simulink model "TENNIS_Ball"  (R2017a)
settings: Solver=ode4  StartTime=0.0  StopTime=1.5  FixedStep=.01  RelTol=1e-7  EnableMultiTasking=on
InitFcn:
  | h =1;        % [m];
  | v0=25;      % [m*s^-1];
  | theta=15;  % [deg];
  | ro=1.29;    % [kg*m^-3];
  | g=9.81;     % [m/s^2]
  | d=.063;     % [m];
  | m=.05;      % [kg];
  | w=20;        % [m*s^-1]; angular velocity of a spinning ball
  | eta=1;        % describes direction(+-) and presence of rotation;
settings Model: Creator=SLE  LastModifiedBy=sulaymon.eshkabilov
settings DataIOCC: Decimation=4  SignalLoggingSaveFormat=ModelDataLogs  SignalLogging=off  SaveTime=off  ReturnWorkspaceOutputs=on
settings OptimizationCC: ExpressionDepthLimit=2147483647  LifeSpan=inf
settings DebuggingCC: UnderspecifiedInitializationDetection=Classic  MergeDetectMultiDrivingBlocksExec=none  SolverPrmCheckMsg=warning  FcnCallInpInsideContextMsg=warning  StateNameClashWarn=warning  SFUnexpectedBacktrackingDiag=warning  SFNoUnconditionalDefaultTransitionDiag=warning  SFExecutionAtInitializationDiag=none
settings HardwareCC: ProdBitPerPointer=32  ProdBitPerSizeT=32  ProdBitPerPtrDiffT=32  ProdLargestAtomicFloat=None  ProdIntDivRoundTo=Undefined  ProdEndianess=Unspecified  ProdWordSize=32  ProdHWDeviceType=32-bit Generic
settings ModelReferenceCC: PropagateSignalLabelsOutOfModel=off
settings RTWCC: GenCodeOnly=on  GenerateReport=on  TLCDebug=on  TLCAssert=on  RTWUseSimCustomCode=on  LaunchReport=on  TargetLang=C++
settings CodeAppCC: ForceParamTrailComments=on  UseSimReservedNames=on
settings GRTTargetCC: TargetLangStandard=C89/C90 (ANSI)  GeneratePreprocessorConditionals=Disable all  CombineOutputUpdateFcns=off  GRTInterface=on
settings ConfigComp: CovMetricSettings=dw  CovHtmlReporting=on  CovSaveCumulativeToWorkspaceVar=on  CovSaveSingleToWorkspaceVar=on  CovExternalEMLEnable=off

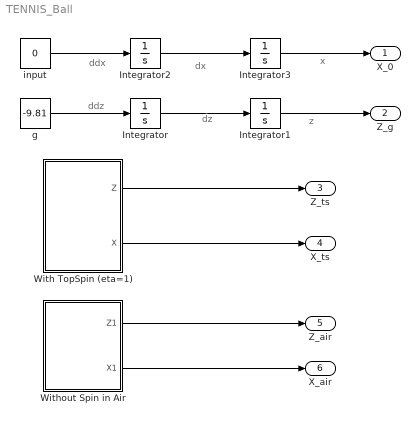
== system TENNIS_Ball ==
  note: dx
  note: x
  note: dz
  note: ddz
  note: z
  note: ddx
  Integrator : Integrator  InitialCondition=25*sin(15*pi/180)
  Integrator1 : Integrator  InitialCondition=1
  Integrator2 : Integrator  InitialCondition=25*cos(15*pi/180)
  Integrator3 : Integrator
  With TopSpin (eta=1) : Subsystem
  Without Spin in Air : Subsystem
  g : Constant  Value=-9.81
  input : Constant  Value=0
  X_0 : Outport
  Z_g : Outport  Port=2
  Z_ts : Outport  Port=3
  X_ts : Outport  Port=4
  Z_air : Outport  Port=5
  X_air : Outport  Port=6
  wires:
  Integrator/1 -> Integrator1/1
  Integrator1/1 -> Z_g/1
  Integrator2/1 -> Integrator3/1
  Integrator3/1 -> X_0/1
  g/1 -> Integrator/1
  input/1 -> Integrator2/1
  With TopSpin (eta=1)/1(Z) -> Z_ts/1
  With TopSpin (eta=1)/2(X) -> X_ts/1
  Without Spin in Air/1(Z1) -> Z_air/1
  Without Spin in Air/2(X1) -> X_air/1

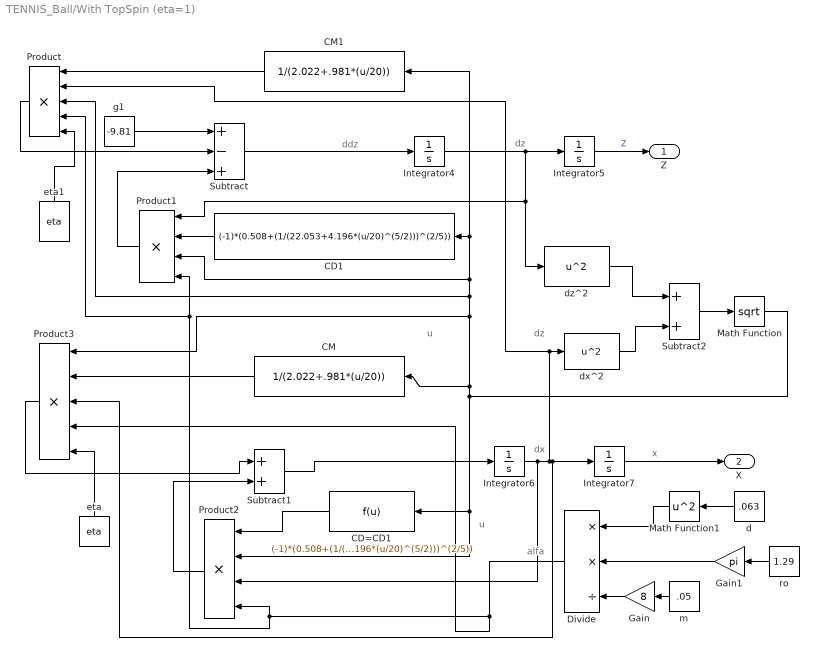
== system TENNIS_Ball/With TopSpin (eta=1) ==
  note: dz
  note: dx
  note: u
  note: u
  note: x
  note: dz
  note: ddz
  note: alfa
  CD1 : Fcn  Expr=(-1)*(0.508+(1/(22.053+4.196*(u/20)^(5/2)))^(2/5))
  CD=CD1 : Fcn  Expr=(-1)*(0.508+(1/(22.053+4.196*(u/20)^(5/2)))^(2/5))
  CM : Fcn  Expr=1/(2.022+.981*(u/20))
  CM1 : Fcn  Expr=1/(2.022+.981*(u/20))
  Divide : Product  Inputs=**/
  Gain : Gain  Gain=8
  Gain1 : Gain  Gain=pi
  Integrator4 : Integrator  InitialCondition=25*sin(15*pi/180)
  Integrator5 : Integrator  InitialCondition=1
  Integrator6 : Integrator  InitialCondition=25*cos(15*pi/180)
  Integrator7 : Integrator
  Math Function : Math  Operator=sqrt  SaturateOnIntegerOverflow=on
  Math Function1 : Math  Operator=square  SaturateOnIntegerOverflow=on
  Product : Product  Inputs=5  RndMeth=Zero
  Product1 : Product  Inputs=4  RndMeth=Zero
  Product2 : Product  Inputs=4  RndMeth=Zero
  Product3 : Product  Inputs=5  RndMeth=Zero
  Subtract : Sum  Inputs=+-+
  Subtract1 : Sum
  Subtract2 : Sum
  d : Constant  Value=.063
  dx^2 : Fcn  Expr=u^2
  dz^2 : Fcn  Expr=u^2
  eta : Constant  Value=eta
  eta1 : Constant  Value=eta
  g1 : Constant  Value=-9.81
  m : Constant  Value=.05
  ro : Constant  Value=1.29
  Z : Outport
  X : Outport  Port=2
  wires:
  Integrator4/1 -> Integrator5/1, dz^2/1, Product1/1
  Integrator5/1 -> Z/1  "Z"
  Integrator6/1 -> Integrator7/1, Product3/3, Product/2, dx^2/1, Product2/3
  Integrator7/1 -> X/1
  Subtract/1 -> Integrator4/1
  Subtract1/1 -> Integrator6/1
  Product2/1 -> Subtract1/2
  CM/1 -> Product3/2
  Product3/1 -> Subtract1/1
  g1/1 -> Subtract/1
  CD1/1 -> Product1/2
  Product1/1 -> Subtract/3
  CM1/1 -> Product/1
  Product/1 -> Subtract/2
  dz^2/1 -> Subtract2/1
  dx^2/1 -> Subtract2/2
  Subtract2/1 -> Math Function/1
  Math Function/1 -> Product1/3, CD1/1, CM1/1, Product/3, Product3/1, CM/1, Product2/2, CD=CD1/1
  Divide/1 -> Product3/4, Product2/4, Product1/4, Product/4
  CD=CD1/1 -> Product2/1
  Gain/1 -> Divide/3
  Gain1/1 -> Divide/2
  Math Function1/1 -> Divide/1
  ro/1 -> Gain1/1
  m/1 -> Gain/1
  d/1 -> Math Function1/1
  eta1/1 -> Product/5
  eta/1 -> Product3/5

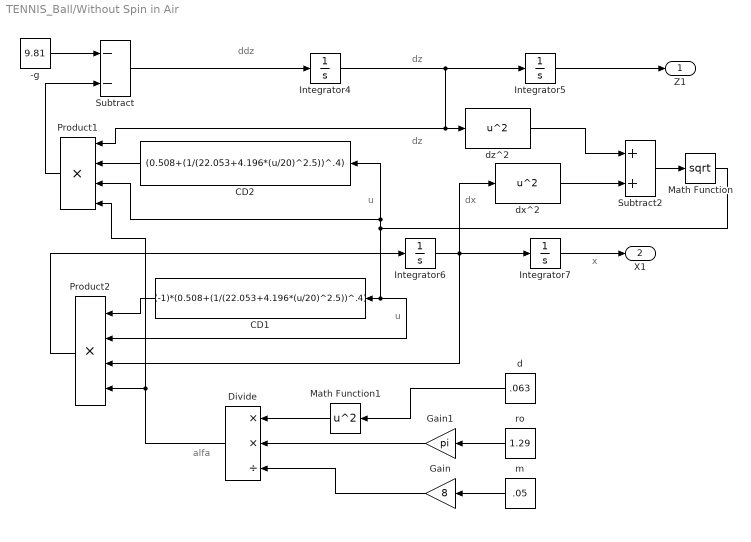
== system TENNIS_Ball/Without Spin in Air ==
  note: dz
  note: dx
  note: u
  note: u
  note: x
  note: dz
  note: ddz
  note: alfa
  -g : Constant  Value=9.81
  CD1 : Fcn  Expr=(-1)*(0.508+(1/(22.053+4.196*(u/20)^2.5))^.4)
  CD2 : Fcn  Expr=(0.508+(1/(22.053+4.196*(u/20)^2.5))^.4)
  Divide : Product  Inputs=**/
  Gain : Gain  Gain=8
  Gain1 : Gain  Gain=pi
  Integrator4 : Integrator  InitialCondition=25*sin(15*pi/180)
  Integrator5 : Integrator  InitialCondition=1
  Integrator6 : Integrator  InitialCondition=25*cos(15*pi/180)
  Integrator7 : Integrator
  Math Function : Math  Operator=sqrt  SaturateOnIntegerOverflow=on
  Math Function1 : Math  Operator=square  SaturateOnIntegerOverflow=on
  Product1 : Product  Inputs=4  RndMeth=Zero
  Product2 : Product  Inputs=4  RndMeth=Zero
  Subtract : Sum  Inputs=--
  Subtract2 : Sum
  d : Constant  Value=.063
  dx^2 : Fcn  Expr=u^2
  dz^2 : Fcn  Expr=u^2
  m : Constant  Value=.05
  ro : Constant  Value=1.29
  Z1 : Outport
  X1 : Outport  Port=2
  wires:
  Integrator4/1 -> Integrator5/1, dz^2/1, Product1/1
  Integrator5/1 -> Z1/1
  Integrator6/1 -> Integrator7/1, Product2/3, dx^2/1
  Integrator7/1 -> X1/1
  Subtract/1 -> Integrator4/1
  Product2/1 -> Integrator6/1
  -g/1 -> Subtract/1
  CD2/1 -> Product1/2
  Product1/1 -> Subtract/2
  dz^2/1 -> Subtract2/1
  dx^2/1 -> Subtract2/2
  Subtract2/1 -> Math Function/1
  Math Function/1 -> Product1/3, CD2/1, Product2/2, CD1/1
  d/1 -> Math Function1/1
  ro/1 -> Gain1/1
  Math Function1/1 -> Divide/1
  Gain1/1 -> Divide/2
  Divide/1 -> Product1/4, Product2/4
  CD1/1 -> Product2/1
  m/1 -> Gain/1
  Gain/1 -> Divide/3
